simulink library "TuneVar"  (R2022b)
settings: Solver=VariableStepAuto  StartTime=0.0  StopTime=10.0  RelTol=1e-3
undefined symbols (not defined in the file or in its folder): activeTunePath, busName, CodeID, outValue, Row, stringParse, TOPs, triggers, Tunes
libraries: $bdroot x3, TOP x1
settings Model: MAModelExclusionFileProxy=C:\work\talariaDev\module\talaria_check_exclusions.xml  Creator=kl13806  LastModifiedBy=kl13806
settings SolverCC: AlgebraicLoopSolver=TrustRegion
settings DebuggingCC: UnconnectedInputMsg=warning  UnconnectedOutputMsg=warning  UnconnectedLineMsg=warning  SFMachineParentedDataDiag=warning  ArithmeticOperatorsInVariantConditions=warning
settings ModelReferenceCC: EnableRefExpFcnMdlSchedulingChecks=on
settings SFSimCC: SimUseLocalCustomCode=off  CustomCodeUndefinedFunction=UseInterfaceOnly
settings RTWCC: RTWUseLocalCustomCode=off  DLArmComputeVersion=19.05
settings CodeAppCC: StateflowObjectComments=on

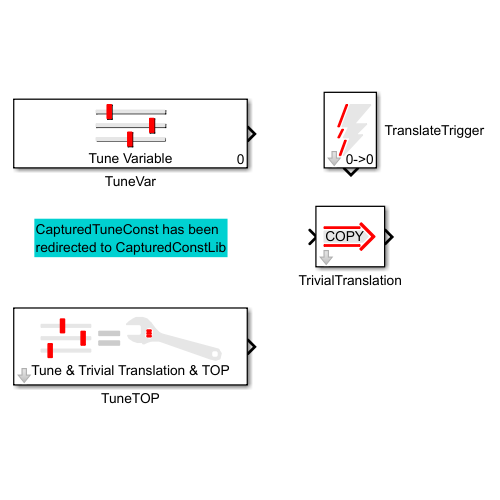
[thumbnail: Simulink's stored preview of the top-level diagram]
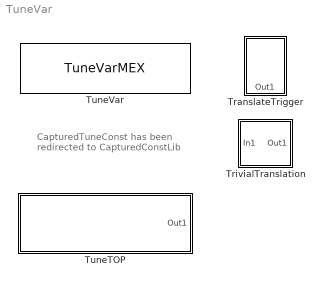
== system TuneVar ==
  note: CapturedTuneConst has been
      | redirected to CapturedConstLib
  TranslateTrigger : Subsystem  mask(Talaria Translate Trigger){TriggerInit=[]}
      mask prompts: TriggerInit "Hidden: MoveFcn redraw"
      mask help: This block generates a function trigger to drive translation blocks
      mask init:
      | [ok,CodeID,Tunes,TOPs] = TranslateTriggerMask.Init(gcbh);
      settings: MoveFcn=TranslateTriggerMask.CB_TriggerInit(gcbh);
      mask Callback TriggerInit: TranslateTriggerMask.CB_TriggerInit(gcbh);
      mask DialogControl ButtonCreateTranslation Prompt: Create sample translation blocks
      mask DialogControl ButtonCreateTranslation Callback: TranslateTriggerMask.CreateEmptyTranslation(gcbh);
      mask DialogControl ButtonClearTOP_Values Prompt: Clear TOP values
      mask DialogControl ButtonClearTOP_Values Callback: TranslateTriggerMask.CB_ClearTOP_Values(gcbh);
      mask DialogControl ButtonResizeTranslator Prompt: Auto-size translator block
      mask DialogControl ButtonResizeTranslator Callback: TranslateTriggerMask.CB_ResizeTranslator(gcbh);
      mask DialogControl ButtonEditData Prompt: Launch "Edit Data" dialog
      mask DialogControl ButtonEditData Callback: TranslateTriggerMask.CB_EditData(gcbh);
      mask DialogControl ButtonEditScript Prompt: Edit script
      mask DialogControl ButtonEditScript Callback: TranslateTriggerMask.CB_EditScript(gcbh);
      mask DialogControl ButtonAutoName Prompt: Rename script In and Out arguments based on blocks
      mask DialogControl ButtonAutoName Callback: TranslateTriggerMask.CB_AutoNameArguments(gcbh);
      mask DialogControl ButtonRunTranslation Prompt:
      | Attempt to run translation right now
      | (Experimental. Ensure successful simulation or data load first)
      mask DialogControl ButtonRunTranslation Callback: TranslateTriggerMask.CB_RunTranslation(gcbh);
      mask DialogControl ErrorContainer Prompt: Error Messages
      mask DialogControl ErrorText Prompt: (Add text here)
      mask DialogControl DependentsText Prompt: (Add text here)
      mask DialogControl SourcesText Prompt: (Add text here)
      mask Display:
      | % retrieve icon definition
      | [path,w,h] = TranslateTriggerMask.Icon();
      | 
      | % retrieve the block's pixel size
      | pos = get(gcbh,'position');
      | bw = pos(3) - pos(1);
      | bh = pos(4) - pos(2);
      | 
      | % draw centered icon
      | xAdj = bw/2 - w/2 + 3;
      | yAdj = bh/2 - h/2;
      | for i=1:length(path)
      |    %path(i).x(end+1) = path(i).x(1);
      |    %path(i).y(end+1) = path(i).y(1);
      |    %plot(path(i).x+xAdj, path(i).y+yAdj);
      |    patch(path(i).x+xAdj, path(i).y+yAdj, path(i).rgb);
      | end
      | 
      | % display a count of how many dependent TOPs we found
      | outCount = 0;
      | inCount = 0;
      | if (exist('TOPs') && ~isempty(TOPs))
      |     outCount = length(strfind(TOPs,',')) + 1;
      | end
      | if (exist('Tunes') && ~isempty(Tunes))
      |     inCount = length(strfind(Tunes,',')) + 1;
      | end
      | inoutTxt = sprintf('%d->%d',inCount,outCount);
      | text(bw-2, 0, inoutTxt, 'horizontalAlignment', 'right', ...
      |      'verticalAlignment', 'bottom');
      | 
      | % show the name or an X
      | if (exist('ok','var') && ok)
      | 	%text(bw*0.5, bh*0.15, 'Translate', 'horizontalAlignment','center');
      | 	patch(0,0,[1 1 1]);
      | 	patch(bw,bh,[1 1 1]);
      | else
      | 	tx=bw*0.03;
      | 	ty=bh*0.03;
      | 	patch([0 tx bw bw-tx], [ty 0 bh-ty bh], [1 0 0]);
      | 	patch([0 bw-tx bw tx], [bh-ty 0 ty bh], [1 0 0]);
      | end
  TrivialTranslation : Subsystem  mask(Talaria Trivial Translation){TriggerInit=[]}
      mask prompts: TriggerInit "Hidden: MoveFcn redraw"
      mask help: A trivial translator connects to a TuneVar on the input side and to a TOP (Target Overlay Parameter) for output. The translator then simply copies the value from TuneVar to TOP with no changes.
      mask init:
      | TrivialTranslationMask.Init(gcbh);
      settings: MoveFcn=TrivialTranslationMask.CB_TriggerInit(gcbh);
      mask Callback TriggerInit: TrivialTranslationMask.CB_TriggerInit(gcbh);
      mask Display:
      | % retrieve icon definition
      | [path,w,h] = TrivialTranslationMask.Icon();
      | 
      | % retrieve the block's pixel size
      | pos = get(gcbh,'position');
      | bw = pos(3) - pos(1);
      | bh = pos(4) - pos(2);
      | 
      | % draw centered icon
      | xAdj = bw/2 - w/2;
      | yAdj = bh/2 - h/2;
      | for i=1:length(path)
      |    patch(path(i).x+xAdj, path(i).y+yAdj, path(i).rgb);
      | end
      | disp('COPY   ');
  TuneTOP : Subsystem  mask(Talaria Trivial Tune TOP){TriggerInit=[55 192 225 248], TopName=, TuneName=, DataTypeOut=single, MaskValue=[1], TunabilityNumber=1, MinValue=[], MaxValue=[], BankNumber=0, PreOverlay=false, PostOverlay=false, UseSameName=on}
      mask prompts: TriggerInit "Hidden: MoveFcn redraw"; TopName "Name:"; TuneName "Name of TuneVar:"; DataTypeOut "Data type:"; MaskValue "Default Value:"; TunabilityNumber "Tunability:"; MinValue "Min Value:"; MaxValue "Max Value:"; BankNumber "Target memory bank number:"; PreOverlay "Requires pre-overlay action:"; PostOverlay "Requires post-overlay action:"; UseSameName "Use same name for tune variable and TOP"
      mask help: The TuneTOP block encapsultes a Target Overlay Parameter, a Tune Variable, and a Trivial Translation between them.
      mask init:
      | [ok,activeTopPath,activeTunePath] = TuneTOP_Mask.Init(gcbh);
      settings: MoveFcn=TuneTOP_Mask.CB_TriggerInit(gcbh);
      mask Callback TriggerInit: TuneTOP_Mask.CB_TriggerInit(gcbh);
      mask TypeOptions TopName: TOP/TopName
      mask TypeOptions TuneName: Tune Variable/TuneName
      mask TypeOptions DataTypeOut: TOP/DataTypeOut
      mask TypeOptions MaskValue: Tune Variable/MaskValue
      mask TypeOptions TunabilityNumber: Tune Variable/TunabilityNumber
      mask Callback TunabilityNumber: TuneVarMask.CB_TunabilityNumber(gcbh);
      mask TypeOptions MinValue: Tune Variable/MinValue
      mask TypeOptions MaxValue: Tune Variable/MaxValue
      mask TypeOptions BankNumber: TOP/BankNumber
      mask TypeOptions PreOverlay: TOP/PreOverlay
      mask TypeOptions PostOverlay: TOP/PostOverlay
      mask Callback UseSameName: TuneTOP_Mask.CB_UseSameName(gcbh);
      mask DialogControl toolPanel Prompt: Tuning Tool Hints
      mask DialogControl DescriptionGroup Prompt: Description
      mask DialogControl EditDescription Prompt: Edit Description
      mask DialogControl EditDescription Callback: TuneTOP_Mask.CB_EditDescription(gcbh);
      mask DialogControl TunabilityText Prompt: Easy: Changes nearly every tuning.
      mask DialogControl AdvancedPanel Prompt: Advanced
      mask DialogControl ConvertToFullTranslation Prompt: Irreversible conversion to full translation
      mask DialogControl ConvertToFullTranslation Callback: TuneTOP_Mask.CB_ConvertToFullTranslation(gcbh);
      mask DialogControl ErrorContainer Prompt: Error Messages
      mask Display:
      | % retrieve icon definition
      | [path,w,h] = TuneTOP_Mask.Icon();
      | 
      | % retrieve the block's pixel size
      | pos = get(gcbh,'position');
      | bw = pos(3) - pos(1);
      | bh = pos(4) - pos(2);
      | 
      | % draw centered icon
      | xAdj = bw/2 - w/2 + 5;
      | yAdj = bh/2 - h/2 + 4;
      | for i=1:length(path)
      | 	patch(path(i).x+xAdj, path(i).y+yAdj, path(i).rgb);
      | end
      | 
      | % show the top name or an X
      | if (exist('ok','var') && ok)
      | 	text(bw*0.5, bh*0.2, activeTopPath, 'horizontalAlignment', 'center');
      | 	patch(0,0,[1 1 1]);
      | 	patch(bw,bh,[1 1 1]);
      | else
      | 	tx=bw*0.03;
      | 	ty=bh*0.03;
      | 	patch([0 tx bw bw-tx], [ty 0 bh-ty bh], [1 0 0]);
      | 	patch([0 bw-tx bw tx], [bh-ty 0 ty bh], [1 0 0]);
      | end
  TuneVar : S-Function  FunctionName=TuneVarMEX  Parameters=activeTunePath,triggers,outValue.Size,outValue.Value,busName,stringParse,VariableDim,0  SFunctionDeploymentMode=off  EnableBusSupport=off  mask(Talaria Tune Variable){TuneName=, MaskValue=[1], SpecifyMaxSize=off, VariableDim=1 (Row), MaxSize=[1 1], TunabilityNumber=1, MinValue=[], MaxValue=[], TriggerInit=[]}
      mask prompts: TuneName "Tune Variable Name:"; MaskValue "Default Value:"; SpecifyMaxSize "Specify Maximum Size"; VariableDim "Variable Dimension"; MaxSize "Max Size:"; TunabilityNumber "Tunability:"; MinValue "Min Value:"; MaxValue "Max Value:"; TriggerInit "Hidden: MoveFcn redraw"
      mask help: Tune variable for calibration of algorithmic content and addressed by system engineering tuning tools. This block outputs a bus signal with .Value and .Size elements. The .Size element specifies the currently supplied dimensions while the .Value element is always sized to hold the maximum possible TuneVar signal determined below. Either explicitly specify max size, or else the supplied default value is assumed to represent the maximum size. See the help for more detail about the dimensions of a TuneVar and how size variance between tunings are handled.
      mask init:
      | [ok,activeTunePath,triggers,outValue,busName,stringParse] = TuneVarMask.Init(gcbh,TuneName,MaskValue,SpecifyMaxSize,MaxSize,VariableDim);
      settings: MoveFcn=TuneVarMask.CB_TriggerInit(gcbh);
      mask Help: TuneVar blocks represent a tune variable that can be changed by tuning tools. In many cases, tune variables are stored directly in ASCII text tune files, but can originate from other sources as well. In a production system application build process or in a production tuning tool, tune variables are changed by invoking the SetTuneVar method of the Talaria Translation Engine DLL  built from the model containing the TuneVar. <br><h2>TuneVar Block Parameters</h2> <b>Tune Variable Name:</b> The name of the tune variable which must be unique within the context of the block's FeaturePath. Notice that the name printed on the block on the modeling canvas is prepended with the FeaturePath discovered within the context of the model. Each FeaturePath block found in the Simulink subsystem hierarchy starting with the TuneVar block in question will contribute to the overall TuneVar instance FeaturePath name for the TuneVar.<br><br> <b>Default Value</b>: This block-specified default value is an evaluated parameter specifying what to feed the tuning translation during the operation of the source model. This value essentially helps to stock the cold-start value for TOPs resulting from translation of the TuneVar. Note that the TalariaTest framework includes methods for temporarily altering this default value for the purposes of testing via the source model. Alternate tune values can be specified to examine the resulting model behavior.<br> Note that TuneVar values have an associated datatypes and dimensions implied by this Default Value. In practice, actual tuning data inherently supports supplying <em>less</em> data than the TuneVar's dimensions would support. See immediately below for more on the TuneVar dimension.<br><br> <b>Specify Max Size:</b> When checked, this control reveals an optional parameter to explicitly specify the maximum dimensions supported by the TuneVar during tuning operations. Instead of automatically determining the maximum size from the Default Value, the explicit maximum size overrides and specifies a larger set of dimensions. Note that the default value and the maximum size still need to make sense relative to each other. A TuneVar cannot specify a default value that is larger than the explicit max size! Similarly, for <em>multi-dimensioned</em> TuneVars the number of dimensions in the default value must match the number of dimensions specified explicitly. During tuning operations, a particular tuning is allowed to provide less data than the TuneVar's maximum size, but this variance takes the form of having fewer rows by default. To change which dimension <em>picks up the slack</em> use the 'Variable Dimension' control. Of course for those TuneVars which are just a vector instead of a matrix (i.e. either a single row or a single column) then the variable size support works for whichever type of vector is present.<br><br> <b>Tuning Tool Hints:</b> The parameters contained in the tuning tool hints section are exactly as described: only hints for use by tuning tools. The values specified here are not enforced. They are only dumped to XML files along with the rest of the for description each TuneVar so that tuning tools and build processes can use or ignore the hints however they deem appropriate. <br><h2>How Do I Use a TuneVar Block?</h2> TuneVar blocks must feed into tuning translation logic. This logic processes one or more TuneVars to result in one or more outbound TOPs (Target Overlay Parameter blocks). Usually, the translation logic is represented by a MATLAB function block, but any logic function-triggered by a TranslateTrigger block should work.<br> For trivial translations where a TuneVar is directly copied into the memory of the embedded target logic (i.e. there is no difference between the TuneVar and the resulting TOP) you may wish to use the TuneTOP block provided by Talaria for this specific purpose. Inside, the TuneTOP block includes a TuneVar, a TOP, and a trivial translation for your convenience.
      mask Callback SpecifyMaxSize: TuneVarMask.CB_SpecifyMaxSize(gcbh);
      mask TypeOptions VariableDim: 1 (Row) | 2 (Column) | 3 (Matrix) | 4 (Cube) | 5 (Tesseract) | 6 (5-cube) | 7 (6-cube)
      mask Callback MaxSize: TuneVarMask.CB_MaxSize(gcbh);
      mask Callback TunabilityNumber: TuneVarMask.CB_TunabilityNumber(gcbh);
      mask Callback TriggerInit: TuneVarMask.CB_TriggerInit(gcbh);
      mask DialogControl toolPanel Prompt: Tuning Tool Hints
      mask DialogControl DescriptionGroup Prompt: Description
      mask DialogControl EditDescription Prompt: Edit Description
      mask DialogControl EditDescription Callback: TuneVarMask.CB_EditDescription(gcbh);
      mask DialogControl ErrorContainer Prompt: Error Messages
      mask Display:
      | % retrieve icon definition
      | [path,w,h] = TuneVarMask.Icon();
      | 
      | % retrieve the block's pixel size
      | pos = get(gcbh,'position');
      | bw = pos(3) - pos(1);
      | bh = pos(4) - pos(2);
      | 
      | % draw centered icon
      | xAdj = bw/2 - w/2;
      | yAdj = bh/2 - h/2 + 6;
      | for i=1:length(path)
      |    path(i).x(end+1) = path(i).x(1);
      |    path(i).y(end+1) = path(i).y(1);
      |    plot(path(i).x+xAdj, path(i).y+yAdj);
      |    patch(path(i).x+xAdj, path(i).y+yAdj, path(i).rgb);
      | end
      | 
      | % display a count of how many dependent translations we found
      | if (exist('triggers','var'))
      |     numTrigs = ~isempty(triggers) + numel(strfind(triggers,','));
      |     text(bw-2, 0, num2str(numTrigs), 'horizontalAlignment', 'right', ...
      |          'verticalAlignment', 'bottom');
      | end
      | % show the name or an X
      | if (exist('ok','var') && ok)
      | 	text(bw*0.5, bh*0.15, activeTunePath, 'horizontalAlignment','center');
      | 	patch(0,0,[1 1 1]);
      | 	patch(bw,bh,[1 1 1]);
      | else
      | 	tx=bw*0.03;
      | 	ty=bh*0.03;
      | 	patch([0 tx bw bw-tx], [ty 0 bh-ty bh], [1 0 0]);
      | 	patch([0 bw-tx bw tx], [bh-ty 0 ty bh], [1 0 0]);
      | end

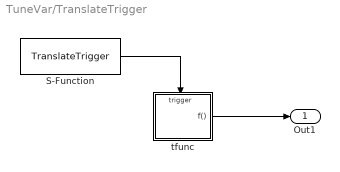
== system TuneVar/TranslateTrigger ==
  S-Function : S-Function  FunctionName=TranslateTrigger  Parameters=CodeID,Tunes,TOPs,0  SFunctionDeploymentMode=off  EnableBusSupport=off
  tfunc : MATLAB Function  TreatAsAtomicUnit=on  RTWFileName=RtcReqRspHandlers
      settings: RTWSystemCode=Nonreusable function
  Out1 : Outport  VectorParamsAs1DForOutWhenUnconnected=off
  wires:
  tfunc/1(f()) -> Out1/1
  S-Function/1 -> tfunc/Trigger

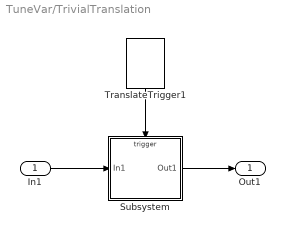
== system TuneVar/TrivialTranslation ==
  In1 : Inport
  Subsystem : Subsystem
  TranslateTrigger1 : $bdroot/TranslateTrigger  TriggerInit=[266 20 304 70]
  Out1 : Outport  VectorParamsAs1DForOutWhenUnconnected=off
  wires:
  In1/1 -> Subsystem/1(In1)
  TranslateTrigger1/1 -> Subsystem/Trigger
  Subsystem/1(Out1) -> Out1/1

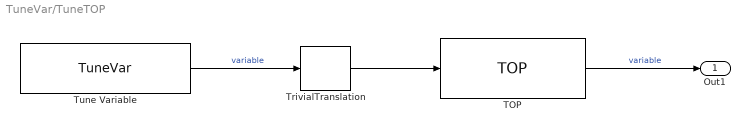
== system TuneVar/TuneTOP ==
  TOP : TOP/TOP  TriggerInit=[440 20 585 80]  DataTypeOut=single  BankNumber=BankNumber  PreOverlay=PreOverlay  PostOverlay=PostOverlay  Role=Automatic
      settings: SourceProductName=Bose Talaria
  TrivialTranslation : $bdroot/TrivialTranslation  TriggerInit=[300 28 350 72]
  Tune Variable : $bdroot/TuneVar  SpecifyMaxSize=off  VariableDim=1 (Row)  MaxSize=[1 1]  TunabilityNumber=1  MinValue=MinValue  MaxValue=MaxValue  TriggerInit=[20 25 190 75]  MaskValue=MaskValue
  Out1 : Outport  VectorParamsAs1DForOutWhenUnconnected=off
  wires:
  TrivialTranslation/1 -> TOP/1
  Tune Variable/1 -> TrivialTranslation/1  "variable"
  TOP/1 -> Out1/1  "variable"

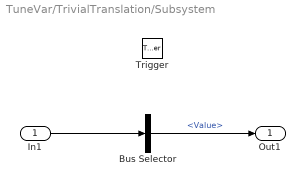
== system TuneVar/TrivialTranslation/Subsystem ==
  In1 : Inport
  Trigger : TriggerPort  TriggerType=function-call  VariantControl=Variant  PortDimensions=1
  Bus Selector : BusSelector  OutputSignals=Value
  Out1 : Outport  VectorParamsAs1DForOutWhenUnconnected=off
  wires:
  Bus Selector/1 -> Out1/1  "<Value>"
  In1/1 -> Bus Selector/1

== matlab function TuneVar/TranslateTrigger/tfunc ==
  events: trigger input FUNCTION_CALL_EVENT; f output FUNCTION_CALL_EVENT
function fcn
% Invoke the function trigger output
f();
